simulink library "aerolibutil"  (Simulink 5.0)
libraries: aerolibutil x3, simulink x3
settings Model: Creator=sgage  LastModifiedBy=sgage  ExtModeAutoUpdateStatusClock=off  TargetHWChar=2  TargetHWWordLengths=8,16,32,32

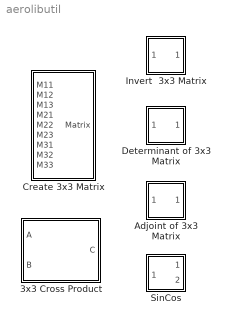
== system aerolibutil ==
  3x3 Cross Product : Subsystem
      mask Type: CrossProduct
      mask Description: Calculate the cross product of two 3-by-1 vectors.
      mask Help: web(asbhelp('3x3crossproduct'));
      mask Display:
      | text(.5,.5,'Cross\nProduct\nC = AxB', ...
      | 	'HorizontalAlignment','Center',...
      | 	'VerticalAlignment','middle')
  Adjoint of 3x3 Matrix : Subsystem
      mask Type: Adjoint of 3x3 matrix
      mask Description: Compute the adjoint matrix for the input matrix.
      mask Help: web(asbhelp);
      mask Display:
      | text(.5,.5,'adj(A)\n(3x3)',...
      | 	'horizontalalignment','center');
  Create 3x3 Matrix : Subsystem
      mask Type: Create 3x3 Matrix
      mask Description:
      | Create a 3-by-3 matrix from nine input values. Each input corresponds to an element of the matrix.
      | 
      | For example, the input labeled A21 is the entry in the second row and first column of the matrix.
      mask Help: web(asbhelp);
      mask Display:
      | port_label('input',1,'A_{11}','texmode','on');
      | port_label('input',2,'A_{12}','texmode','on');
      | port_label('input',3,'A_{13}','texmode','on');
      | port_label('input',4,'A_{21}','texmode','on');
      | port_label('input',5,'A_{22}','texmode','on');
      | port_label('input',6,'A_{23}','texmode','on');
      | port_label('input',7,'A_{31}','texmode','on');
      | port_label('input',8,'A_{32}','texmode','on');
      | port_label('input',9,'A_{33}','texmode','on');
      | port_label('output',1,'A','texmode','on');
  Determinant of 3x3 Matrix : Subsystem
      mask Type: Determinant of 3x3 Matrix
      mask Description: Compute the determinant of 3x3 matrix.
      mask Help: web(asbhelp);
      mask Display:
      | text(.5,.5,'det(A)\n(3x3)',...
      | 	'horizontalalignment','center');
  Invert  3x3 Matrix : Subsystem
      mask Type: Invert 3x3 Matrix
      mask Description: Compute the inverse of 3-by-3 matrix using determinant formula.
      mask Help: web(asbhelp);
      mask Display:
      | text(.5,.675,'A^{-1}','texmode','on',...
      | 	'horizontalalignment','center');
      | text(.5,.325,'(3x3)','texmode','on',...
      | 	'horizontalalignment','center');
  SinCos : Subsystem
      mask Type: SinCos
      mask Description: Compute the sine and cosine of input, u. u is in radians.
      mask Help: web(asbhelp);
      mask Display:
      | port_label('output',1,'sin(u)','texmode','on');
      | port_label('output',2,'cos(u)','texmode','on');

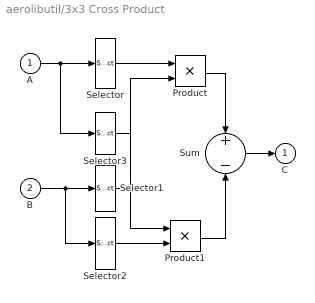
== system aerolibutil/3x3 Cross Product ==
  A : Inport
  B : Inport  Port=2
  Product : Product  SaturateOnIntegerOverflow=on  InputSameDT=on
  Product1 : Product  SaturateOnIntegerOverflow=on  InputSameDT=on
  Selector : Selector  Elements=[2 3 1]  InputPortWidth=3
  Selector1 : Selector  Elements=[3 1 2]  InputPortWidth=3
  Selector2 : Selector  Elements=[2 3 1]  InputPortWidth=3
  Selector3 : Selector  Elements=[3 1 2]  InputPortWidth=3
  Sum : Sum  Inputs=+|-  SaturateOnIntegerOverflow=on  InputSameDT=on
  C : Outport  InitialOutput=0
  wires:
  Selector3/1 -> Product1/1
  Selector2/1 -> Product1/2
  Product1/1 -> Sum/2
  Selector1/1 -> Product/2
  Product/1 -> Sum/1
  A/1 -> Selector3/1, Selector/1
  Selector/1 -> Product/1
  B/1 -> Selector2/1, Selector1/1
  Sum/1 -> C/1

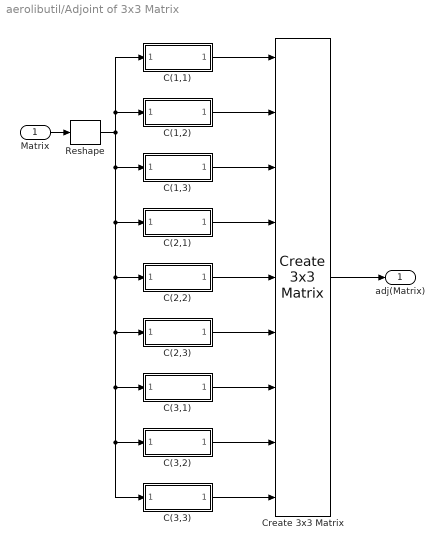
== system aerolibutil/Adjoint of 3x3 Matrix ==
  Matrix : Inport
  C(1,1) : Subsystem
  C(1,2) : Subsystem
  C(1,3) : Subsystem
  C(2,1) : Subsystem
  C(2,2) : Subsystem
  C(2,3) : Subsystem
  C(3,1) : Subsystem
  C(3,2) : Subsystem
  C(3,3) : Subsystem
  Create 3x3 Matrix : aerolibutil/Create 3x3 Matrix
  Reshape : simulink/Math Operations/Reshape  OutputDimensionality=Column vector  OutputDimensions=[1,1]
  adj(Matrix) : Outport
  wires:
  Reshape/1 -> C(1,1)/1(Matrix), C(1,2)/1(Matrix), C(3,3)/1(Matrix), C(3,2)/1(Matrix), C(3,1)/1(Matrix), C(2,3)/1(Matrix), C(2,2)/1(Matrix), C(2,1)/1(Matrix), C(1,3)/1(Matrix)
  C(1,2)/1(C(1,2)) -> Create 3x3 Matrix/2
  C(1,3)/1(C(1,3)) -> Create 3x3 Matrix/3
  C(2,1)/1(C(2,1)) -> Create 3x3 Matrix/4
  C(2,3)/1(C(2,3)) -> Create 3x3 Matrix/6
  C(3,1)/1(C(3,1)) -> Create 3x3 Matrix/7
  C(3,2)/1(C(3,2)) -> Create 3x3 Matrix/8
  Create 3x3 Matrix/1 -> adj(Matrix)/1
  C(3,3)/1(C(3,3)) -> Create 3x3 Matrix/9
  C(2,2)/1(C(2,2)) -> Create 3x3 Matrix/5
  C(1,1)/1(C(1,1)) -> Create 3x3 Matrix/1
  Matrix/1 -> Reshape/1

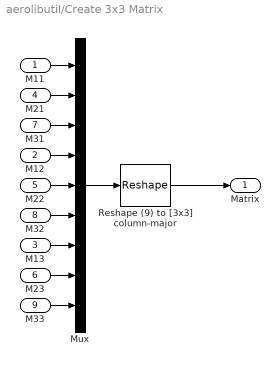
== system aerolibutil/Create 3x3 Matrix ==
  M11 : Inport
  M12 : Inport  Port=2
  M13 : Inport  Port=3
  M21 : Inport  Port=4
  M22 : Inport  Port=5
  M23 : Inport  Port=6
  M31 : Inport  Port=7
  M32 : Inport  Port=8
  M33 : Inport  Port=9
  Mux : Mux  Inputs=9
  Reshape (9) to [3x3] column-major : simulink/Math Operations/Reshape  OutputDimensionality=Customize  OutputDimensions=[3,3]
  Matrix : Outport
  wires:
  Mux/1 -> Reshape (9) to [3x3] column-major/1
  M11/1 -> Mux/1
  M21/1 -> Mux/2
  M31/1 -> Mux/3
  M12/1 -> Mux/4
  M22/1 -> Mux/5
  Reshape (9) to [3x3] column-major/1 -> Matrix/1
  M32/1 -> Mux/6
  M13/1 -> Mux/7
  M23/1 -> Mux/8
  M33/1 -> Mux/9

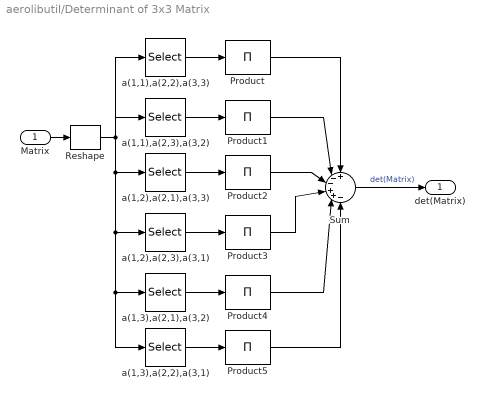
== system aerolibutil/Determinant of 3x3 Matrix ==
  Matrix : Inport
  Product{,1..5} (6 alike) : Product  Inputs=1  SaturateOnIntegerOverflow=on
  Reshape : simulink/Math Operations/Reshape  OutputDimensionality=Column vector  OutputDimensions=[1,1]
  Sum : Sum  Inputs=+--++-  SaturateOnIntegerOverflow=on
  a(1,1),a(2,2),a(3,3) : Selector  Elements=[1 5 9]  InputPortWidth=9
  a(1,1),a(2,3),a(3,2) : Selector  Elements=[1 6 8]  InputPortWidth=9
  a(1,2),a(2,1),a(3,3) : Selector  Elements=[2 4 9]  InputPortWidth=9
  a(1,2),a(2,3),a(3,1) : Selector  Elements=[3 4 8]  InputPortWidth=9
  a(1,3),a(2,1),a(3,2) : Selector  Elements=[2 6 7]  InputPortWidth=9
  a(1,3),a(2,2),a(3,1) : Selector  Elements=[3 5 7]  InputPortWidth=9
  det(Matrix) : Outport
  wires:
  Reshape/1 -> a(1,3),a(2,2),a(3,1)/1, a(1,3),a(2,1),a(3,2)/1, a(1,2),a(2,3),a(3,1)/1, a(1,2),a(2,1),a(3,3)/1, a(1,1),a(2,3),a(3,2)/1, a(1,1),a(2,2),a(3,3)/1
  Sum/1 -> det(Matrix)/1  "det(Matrix)"
  Matrix/1 -> Reshape/1
  Product5/1 -> Sum/6
  Product4/1 -> Sum/5
  Product3/1 -> Sum/4
  Product2/1 -> Sum/3
  Product1/1 -> Sum/2
  Product/1 -> Sum/1
  a(1,3),a(2,2),a(3,1)/1 -> Product5/1
  a(1,3),a(2,1),a(3,2)/1 -> Product4/1
  a(1,2),a(2,3),a(3,1)/1 -> Product3/1
  a(1,2),a(2,1),a(3,3)/1 -> Product2/1
  a(1,1),a(2,3),a(3,2)/1 -> Product1/1
  a(1,1),a(2,2),a(3,3)/1 -> Product/1

== system aerolibutil/Invert  3x3 Matrix ==
  Matrix : Inport
  Adjoint of 3x3 Matrix : aerolibutil/Adjoint of 3x3 Matrix
  Assertion : Assertion  AssertionFailFcn="disp('Matrix is singular.  No matrix inverse.')"
  Determinant of 3x3 Matrix : aerolibutil/Determinant of 3x3 Matrix
  Product : Product  Inputs=/*  SaturateOnIntegerOverflow=on
  Matrix' : Outport
  wires:
  Matrix/1 -> Determinant of 3x3 Matrix/1, Adjoint of 3x3 Matrix/1
  Determinant of 3x3 Matrix/1 -> Assertion/1, Product/1
  Adjoint of 3x3 Matrix/1 -> Product/2
  Product/1 -> Matrix'/1

== system aerolibutil/SinCos ==
  theta : Inport
  cosine : Trigonometry  Operator=cos
  sine : Trigonometry
  sin(theta) : Outport
  cos(theta) : Outport  Port=2
  wires:
  theta/1 -> sine/1, cosine/1
  sine/1 -> sin(theta)/1
  cosine/1 -> cos(theta)/1

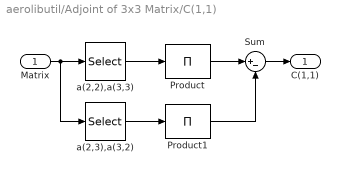
== system aerolibutil/Adjoint of 3x3 Matrix/C(1,1) ==
  Matrix : Inport
  Product : Product  Inputs=1  SaturateOnIntegerOverflow=on
  Product1 : Product  Inputs=1  SaturateOnIntegerOverflow=on
  Sum : Sum  Inputs=|+-  SaturateOnIntegerOverflow=on
  a(2,2),a(3,3) : Selector  Elements=[5 9]  InputPortWidth=9
  a(2,3),a(3,2) : Selector  Elements=[6 8]  InputPortWidth=9
  C(1,1) : Outport
  wires:
  a(2,2),a(3,3)/1 -> Product/1
  a(2,3),a(3,2)/1 -> Product1/1
  Product/1 -> Sum/1
  Product1/1 -> Sum/2
  Sum/1 -> C(1,1)/1
  Matrix/1 -> a(2,2),a(3,3)/1, a(2,3),a(3,2)/1

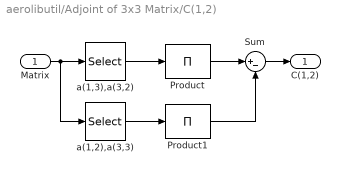
== system aerolibutil/Adjoint of 3x3 Matrix/C(1,2) ==
  Matrix : Inport
  Product : Product  Inputs=1  SaturateOnIntegerOverflow=on
  Product1 : Product  Inputs=1  SaturateOnIntegerOverflow=on
  Sum : Sum  Inputs=|+-  SaturateOnIntegerOverflow=on
  a(1,2),a(3,3) : Selector  Elements=[4 9]  InputPortWidth=9
  a(1,3),a(3,2) : Selector  Elements=[6 7]  InputPortWidth=9
  C(1,2) : Outport
  wires:
  Matrix/1 -> a(1,2),a(3,3)/1, a(1,3),a(3,2)/1
  Sum/1 -> C(1,2)/1
  Product1/1 -> Sum/2
  Product/1 -> Sum/1
  a(1,2),a(3,3)/1 -> Product1/1
  a(1,3),a(3,2)/1 -> Product/1

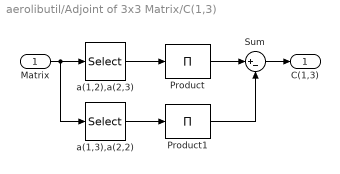
== system aerolibutil/Adjoint of 3x3 Matrix/C(1,3) ==
  Matrix : Inport
  Product : Product  Inputs=1  SaturateOnIntegerOverflow=on
  Product1 : Product  Inputs=1  SaturateOnIntegerOverflow=on
  Sum : Sum  Inputs=|+-  SaturateOnIntegerOverflow=on
  a(1,2),a(2,3) : Selector  Elements=[4 8]  InputPortWidth=9
  a(1,3),a(2,2) : Selector  Elements=[5 7]  InputPortWidth=9
  C(1,3) : Outport
  wires:
  a(1,2),a(2,3)/1 -> Product/1
  a(1,3),a(2,2)/1 -> Product1/1
  Product/1 -> Sum/1
  Product1/1 -> Sum/2
  Sum/1 -> C(1,3)/1
  Matrix/1 -> a(1,3),a(2,2)/1, a(1,2),a(2,3)/1

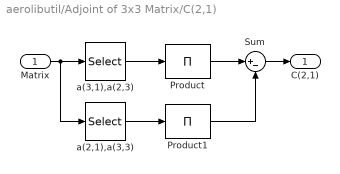
== system aerolibutil/Adjoint of 3x3 Matrix/C(2,1) ==
  Matrix : Inport
  Product : Product  Inputs=1  SaturateOnIntegerOverflow=on
  Product1 : Product  Inputs=1  SaturateOnIntegerOverflow=on
  Sum : Sum  Inputs=|+-  SaturateOnIntegerOverflow=on
  a(2,1),a(3,3) : Selector  Elements=[2 9]  InputPortWidth=9
  a(3,1),a(2,3) : Selector  Elements=[3 8]  InputPortWidth=9
  C(2,1) : Outport
  wires:
  Matrix/1 -> a(2,1),a(3,3)/1, a(3,1),a(2,3)/1
  Sum/1 -> C(2,1)/1
  Product1/1 -> Sum/2
  Product/1 -> Sum/1
  a(2,1),a(3,3)/1 -> Product1/1
  a(3,1),a(2,3)/1 -> Product/1

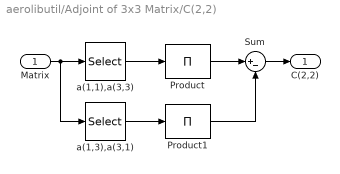
== system aerolibutil/Adjoint of 3x3 Matrix/C(2,2) ==
  Matrix : Inport
  Product : Product  Inputs=1  SaturateOnIntegerOverflow=on
  Product1 : Product  Inputs=1  SaturateOnIntegerOverflow=on
  Sum : Sum  Inputs=|+-  SaturateOnIntegerOverflow=on
  a(1,1),a(3,3) : Selector  Elements=[1 9]  InputPortWidth=9
  a(1,3),a(3,1) : Selector  Elements=[3 7]  InputPortWidth=9
  C(2,2) : Outport
  wires:
  a(1,1),a(3,3)/1 -> Product/1
  a(1,3),a(3,1)/1 -> Product1/1
  Product/1 -> Sum/1
  Product1/1 -> Sum/2
  Sum/1 -> C(2,2)/1
  Matrix/1 -> a(1,1),a(3,3)/1, a(1,3),a(3,1)/1

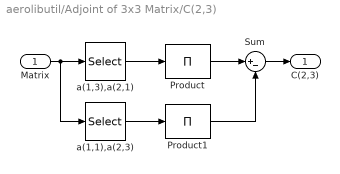
== system aerolibutil/Adjoint of 3x3 Matrix/C(2,3) ==
  Matrix : Inport
  Product : Product  Inputs=1  SaturateOnIntegerOverflow=on
  Product1 : Product  Inputs=1  SaturateOnIntegerOverflow=on
  Sum : Sum  Inputs=|+-  SaturateOnIntegerOverflow=on
  a(1,1),a(2,3) : Selector  Elements=[1 8]  InputPortWidth=9
  a(1,3),a(2,1) : Selector  Elements=[2 7]  InputPortWidth=9
  C(2,3) : Outport
  wires:
  Matrix/1 -> a(1,1),a(2,3)/1, a(1,3),a(2,1)/1
  Sum/1 -> C(2,3)/1
  Product1/1 -> Sum/2
  Product/1 -> Sum/1
  a(1,1),a(2,3)/1 -> Product1/1
  a(1,3),a(2,1)/1 -> Product/1

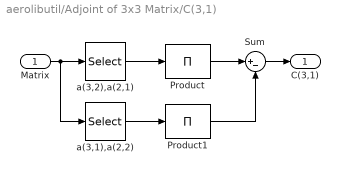
== system aerolibutil/Adjoint of 3x3 Matrix/C(3,1) ==
  Matrix : Inport
  Product : Product  Inputs=1  SaturateOnIntegerOverflow=on
  Product1 : Product  Inputs=1  SaturateOnIntegerOverflow=on
  Sum : Sum  Inputs=|+-  SaturateOnIntegerOverflow=on
  a(3,1),a(2,2) : Selector  Elements=[3 5]  InputPortWidth=9
  a(3,2),a(2,1) : Selector  Elements=[2 6]  InputPortWidth=9
  C(3,1) : Outport
  wires:
  a(3,2),a(2,1)/1 -> Product/1
  a(3,1),a(2,2)/1 -> Product1/1
  Product/1 -> Sum/1
  Product1/1 -> Sum/2
  Sum/1 -> C(3,1)/1
  Matrix/1 -> a(3,2),a(2,1)/1, a(3,1),a(2,2)/1

== system aerolibutil/Adjoint of 3x3 Matrix/C(3,2) ==
  Matrix : Inport
  Product : Product  Inputs=1  SaturateOnIntegerOverflow=on
  Product1 : Product  Inputs=1  SaturateOnIntegerOverflow=on
  Sum : Sum  Inputs=|+-  SaturateOnIntegerOverflow=on
  a(1,1),a(3,2) : Selector  Elements=[1 6]  InputPortWidth=9
  a(1,2),a(3,1) : Selector  Elements=[3 4]  InputPortWidth=9
  C(3,2) : Outport
  wires:
  Matrix/1 -> a(1,1),a(3,2)/1, a(1,2),a(3,1)/1
  Sum/1 -> C(3,2)/1
  Product1/1 -> Sum/2
  Product/1 -> Sum/1
  a(1,1),a(3,2)/1 -> Product1/1
  a(1,2),a(3,1)/1 -> Product/1

== system aerolibutil/Adjoint of 3x3 Matrix/C(3,3) ==
  Matrix : Inport
  Product : Product  Inputs=1  SaturateOnIntegerOverflow=on
  Product1 : Product  Inputs=1  SaturateOnIntegerOverflow=on
  Sum : Sum  Inputs=|+-  SaturateOnIntegerOverflow=on
  a(1,1),a(2,2) : Selector  Elements=[1 5]  InputPortWidth=9
  a(1,2),a(2,1) : Selector  Elements=[2 4]  InputPortWidth=9
  C(3,3) : Outport
  wires:
  Matrix/1 -> a(1,2),a(2,1)/1, a(1,1),a(2,2)/1
  Sum/1 -> C(3,3)/1
  Product1/1 -> Sum/2
  Product/1 -> Sum/1
  a(1,2),a(2,1)/1 -> Product1/1
  a(1,1),a(2,2)/1 -> Product/1
